simulink model "Simulink_model_problem_5_1"  (R2023b)
settings: Solver=VariableStepAuto  StartTime=0.0  StopTime=20  FixedStep=0.001  RelTol=1e-3
settings Model: Creator=sarth  LastModifiedBy=sarth

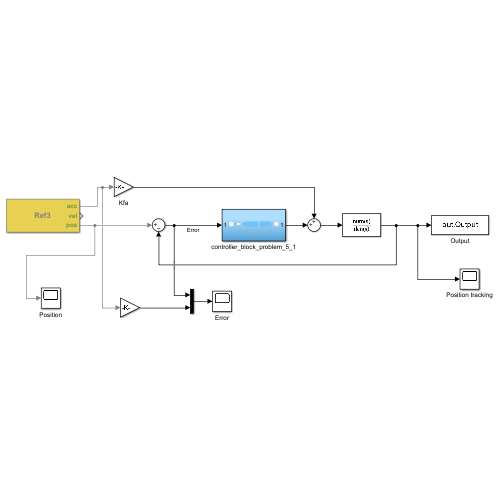
[thumbnail: Simulink's stored preview of the top-level diagram]
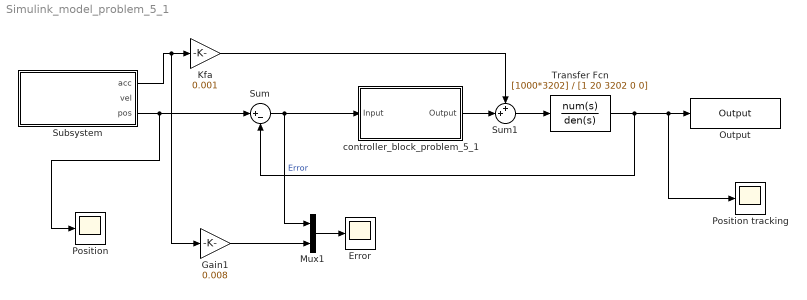
== system Simulink_model_problem_5_1 ==
  Error : Scope
  Gain1 : Gain  Gain=0.008  SaturateOnIntegerOverflow=on  OutDataTypeStr=Inherit: Same as input  ParamDataTypeStr=Inherit: Same as input
  Kfa : Gain  Gain=0.001
  Mux1 : Mux  Inputs=2
  Output : ToWorkspace  VariableName=Output  SaveFormat=Timeseries  SampleTime=-1
  Position : Scope
  Position tracking : Scope
  Subsystem : Subsystem  mask(Ref3){}
      settings: OpenFcn=r3g_main
      mask Display: disp('Ref3');
  Sum : Sum  Inputs=|+-
  Sum1 : Sum  Inputs=++|
  Transfer Fcn : TransferFcn  Numerator=[1000*3202]  Denominator=[1 20 3202 0 0]
  controller_block_problem_5_1 : Subsystem
  wires:
  Subsystem/3(pos) -> Sum/1, Position/1
  Sum/1 -> Mux1/1, controller_block_problem_5_1/1(Input)  "Error"
  Transfer Fcn/1 -> Position tracking/1, Output/1, Sum/2
  Kfa/1 -> Sum1/1
  controller_block_problem_5_1/1(Output) -> Sum1/2
  Sum1/1 -> Transfer Fcn/1
  Gain1/1 -> Mux1/2
  Mux1/1 -> Error/1
  Subsystem/1(acc) -> Gain1/1, Kfa/1

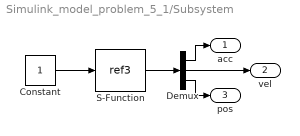
== system Simulink_model_problem_5_1/Subsystem ==
  Constant : Constant
  Demux : Demux  Outputs=3
      settings: DisplayOption=none
  S-Function : S-Function  FunctionName=ref3  Parameters=ref_part  SFunctionDeploymentMode=off  EnableBusSupport=off
      settings: OpenFcn=global ref_part; r3g_main
  acc : Outport
  vel : Outport  Port=2
  pos : Outport  Port=3
  wires:
  Constant/1 -> S-Function/1
  S-Function/1 -> Demux/1
  Demux/1 -> acc/1
  Demux/2 -> vel/1
  Demux/3 -> pos/1

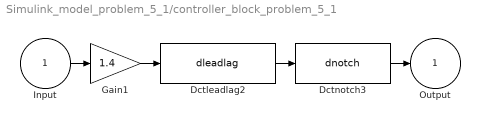
== system Simulink_model_problem_5_1/controller_block_problem_5_1 ==
  Input : Inport
  Dctleadlag2 : S-Function  FunctionName=dleadlag  Parameters=f_num, f_den, 0.001  SFunctionDeploymentMode=off  EnableBusSupport=off  mask(dctools){f_num=6, f_den=500}
      mask prompts: f_num "Zero [Hz]"; f_den "Pole [Hz]"
      mask help: This block implements a discrete time leadlag filter.
      mask Display: disp('DCT leadlag')
  Dctnotch3 : S-Function  FunctionName=dnotch  Parameters=f_num, b_num, f_den, b_den, 0.001  SFunctionDeploymentMode=off  EnableBusSupport=off  mask(dctools){f_num=8.7, b_num=0.25, f_den=40, b_den=0.5}
      mask prompts: f_num "Zero [Hz]"; b_num "Damping zero [-]"; f_den "Pole [Hz]"; b_den "Damping pole [-]"
      mask help: This block implements a dicrete time 2nd order notch filter.
      mask Display: disp('DCT notch')
  Gain1 : Gain  Gain=1.4
  Output : Outport
  wires:
  Input/1 -> Gain1/1
  Gain1/1 -> Dctleadlag2/1
  Dctleadlag2/1 -> Dctnotch3/1
  Dctnotch3/1 -> Output/1
